simulink model "Tank_cilindrico_desc_base"  (R2018b)
settings: Solver=VariableStepAuto  StartTime=0.0  StopTime=150.0  RelTol=1e-3
undefined symbols (not defined in the file or in its folder): sigbuilder_block
settings Model: Creator=joseb  LastModifiedBy=joseb

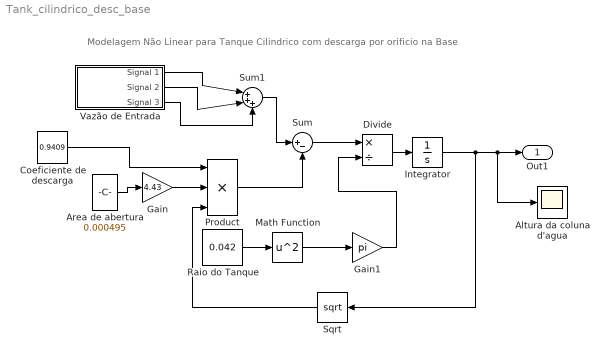
== system Tank_cilindrico_desc_base ==
  note: Modelagem Não Linear para Tanque Cilindrico com descarga por orificio na Base
  Altura da coluna d'agua : Scope
  Area de abertura : Constant  Value=0.000495
  Coeficiente de descarga : Constant  Value=0.9409
  Divide : Product  Inputs=*/
  Gain : Gain  Gain=4.43
  Gain1 : Gain  Gain=pi
  Integrator : Integrator
  Math Function : Math  Operator=square  SaturateOnIntegerOverflow=on
  Product : Product  Inputs=3
  Raio do Tanque : Constant  Value=0.042
  Sqrt : Sqrt  SaturateOnIntegerOverflow=on
  Sum : Sum  Inputs=|+-
  Sum1 : Sum  Inputs=|+++
  Vazão de Entrada : Subsystem  Tag=STV Subsys  LoadFcn=sigbuilder_block('load',[1440 162 1152 590.25 ]);  StartFcn=sigbuilder_block('start');  StopFcn=sigbuilder_block('stop');  ClipboardFcn=sigbuilder_block('clipboard');  mask(Sigbuilder block){tuvar=[0:10]}
      mask help: Simulink:masks:SigbuilderBlock_MD
      mask init:
      | if ~strcmp(get_param(bdroot(gcbh),'SimulationStatus'),'stopped') tuvar = sigbuilder_block('maskInit'); end
      settings: CopyFcn=sigbuilder_block('copy');  DeleteFcn=sigbuilder_block('delete');  ModelCloseFcn=sigbuilder_block('modelClose');  PreSaveFcn=sigbuilder_block('preSave');  PauseFcn=sigbuilder_block('pause');  ContinueFcn=sigbuilder_block('continue');  NameChangeFcn=sigbuilder_block('namechange');  OpenFcn=sigbuilder_block('open',[5.4 0 1141.2 552.6 ]);  CloseFcn=sigbuilder_block('close');
      mask Display: plot(0, 0, 100, 100,[2, 2, 32, 32, 2], [68, 8, 8, 68, 68],[32, 2], [38, 38], [32, 19, 2],[53, 60, 44], [32, 17, 17, 2],[16, 16, 31, 31]);txt = getActiveGroup(gcbh);text(2, 100, txt,'verticalAlignment', 'top');
  Out1 : Outport
  wires:
  Integrator/1 -> Sqrt/1, Altura da coluna d'agua/1, Out1/1
  Area de abertura/1 -> Gain/1
  Sqrt/1 -> Product/3
  Product/1 -> Sum/2
  Divide/1 -> Integrator/1
  Sum/1 -> Divide/1
  Gain1/1 -> Divide/2
  Raio do Tanque/1 -> Math Function/1
  Math Function/1 -> Gain1/1
  Gain/1 -> Product/2
  Coeficiente de descarga/1 -> Product/1
  Sum1/1 -> Sum/1
  Vazão de Entrada/1(Signal 1) -> Sum1/1
  Vazão de Entrada/2(Signal 2) -> Sum1/2
  Vazão de Entrada/3(Signal 3) -> Sum1/3

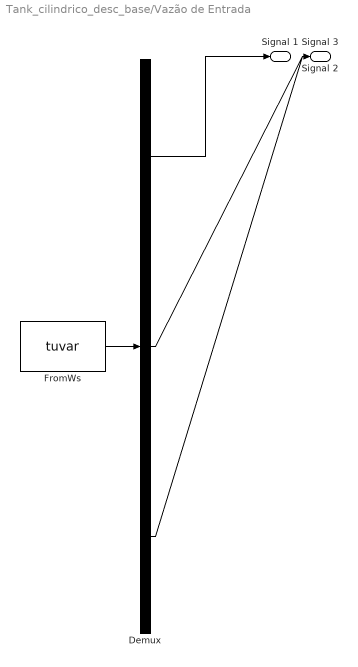
== system Tank_cilindrico_desc_base/Vazão de Entrada ==
  Demux : Demux  Tag=STV Demux  Outputs=3
  FromWs : FromWorkspace  Tag=STV FromWs  VariableName=tuvar  SampleTime=0
      SigBuilderData=|
      | common.afterFinalStr = 'Extrapolate'
      | common.sampleTime = 0
      | dataSet.timeRange = [0 150]
      | dataSet.name = 'Group 1'
      | sbobj.Groups.Name = 'Group 1'
      | sbobj.Groups.Signals(1).Name = 'Signal 1'
      | sbobj.Groups.Signals(1).XData = [0 2.5 2.5 50 50 150]
      | sbobj.Groups.Signals(1).YData = [0 0 0.001 0.001 0 0]
      | sbobj.Groups.Signals(2).Name = 'Signal 2'
      | sbobj.Groups.Signals(2).XData = [0 50 50 100 100 150]
      | sbobj.Groups.Signals(2).YData = [0 0 0.0012 0.0012 0 0]
      | sbobj.Groups.Signals(3).Name = 'Signal 3'
      | sbobj.Groups.Signals(3).XData = [0 100 100 131.5 131.5 150]
      | sbobj.Groups.Signals(3).YData = [0 0 0.0016 0.0016 0 0]
      | sbobj.Groups.TimeRange = [0 150]
  Signal 1 : Outport  Tag=STV Outport
  Signal 2 : Outport  Tag=STV Outport  Port=2
  Signal 3 : Outport  Tag=STV Outport  Port=3
  wires:
  Demux/1 -> Signal 1/1
  FromWs/1 -> Demux/1
  Demux/2 -> Signal 2/1
  Demux/3 -> Signal 3/1
